simulink model "linearTFy2y"  (Simulink 7.7)
settings: Solver=ode45  StartTime=0.0  StopTime=700  RelTol=1e-3
values from neighbouring files (symbols this model uses):
  QT =     [FaseMinima.mat]    (also in FaseNaoMinima.mat; FaseNaoMinimaMudandoApenasGama.mat; settup.m = dynamics())
settings Model: Creator=Arthur  LastModifiedBy=Arthur

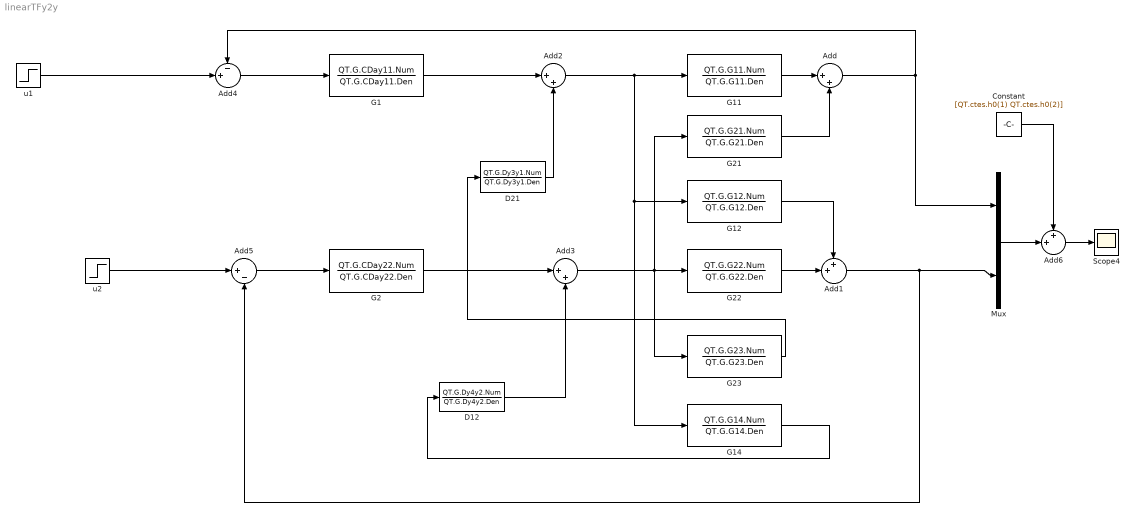
== system linearTFy2y ==
  Add : Sum  Inputs=|++
  Add1 : Sum  Inputs=++|
  Add2 : Sum  Inputs=|++
  Add3 : Sum  Inputs=|++
  Add4 : Sum  Inputs=-+|
  Add5 : Sum  Inputs=|+-
  Add6 : Sum  Inputs=++|
  Constant : Constant  Value=[QT.ctes.h0(1) QT.ctes.h0(2)]
  D12 : TransferFcn  Numerator=QT.G.Dy4y2.Num  Denominator=QT.G.Dy4y2.Den
  D21 : TransferFcn  Numerator=QT.G.Dy3y1.Num  Denominator=QT.G.Dy3y1.Den
  G1 : TransferFcn  Numerator=QT.G.CDay11.Num  Denominator=QT.G.CDay11.Den
  G11 : TransferFcn  Numerator=QT.G.G11.Num  Denominator=QT.G.G11.Den
  G12 : TransferFcn  Numerator=QT.G.G12.Num  Denominator=QT.G.G12.Den
  G14 : TransferFcn  Numerator=QT.G.G14.Num  Denominator=QT.G.G14.Den
  G2 : TransferFcn  Numerator=QT.G.CDay22.Num  Denominator=QT.G.CDay22.Den
  G21 : TransferFcn  Numerator=QT.G.G21.Num  Denominator=QT.G.G21.Den
  G22 : TransferFcn  Numerator=QT.G.G22.Num  Denominator=QT.G.G22.Den
  G23 : TransferFcn  Numerator=QT.G.G23.Num  Denominator=QT.G.G23.Den
  Mux : Mux  Inputs=2
  Scope4 : Scope
      settings: TimeRange=10  SaveName=Simulado
  u1 : Step  Time=200  SampleTime=0
  u2 : Step  Time=500  SampleTime=0
  wires:
  G11/1 -> Add/1
  G21/1 -> Add/2
  G22/1 -> Add1/2
  G12/1 -> Add1/1
  Add/1 -> Mux/1, Add4/1
  Add2/1 -> G11/1, G12/1, G14/1
  Add3/1 -> G22/1, G23/1, G21/1
  G14/1 -> D12/1
  G23/1 -> D21/1
  Add1/1 -> Mux/2, Add5/2
  Add4/1 -> G1/1
  Add5/1 -> G2/1
  u1/1 -> Add4/2
  u2/1 -> Add5/1
  D12/1 -> Add3/2
  D21/1 -> Add2/2
  G1/1 -> Add2/1
  G2/1 -> Add3/1
  Mux/1 -> Add6/2
  Add6/1 -> Scope4/1
  Constant/1 -> Add6/1
